simulink model "arduino_lab"  (R2017a)
settings: Solver=VariableStepAuto  StartTime=0.0  StopTime=500  RelTol=1e-3  EnableMultiTasking=on
StartFcn:
  | clear all
libraries: realtime_pacer_lib x1
settings Model: Creator=johnh  LastModifiedBy=John Hedengren
settings OptimizationCC: LifeSpan=inf
settings DebuggingCC: SFUnexpectedBacktrackingDiag=warning  SFNoUnconditionalDefaultTransitionDiag=warning  SFExecutionAtInitializationDiag=none
settings GRTTargetCC: TargetLangStandard=C89/C90 (ANSI)  GeneratePreprocessorConditionals=Disable all
settings ConfigComp: CovMetricSettings=dw  CovHtmlReporting=on  CovSaveCumulativeToWorkspaceVar=on  CovSaveSingleToWorkspaceVar=on  CovExternalEMLEnable=off

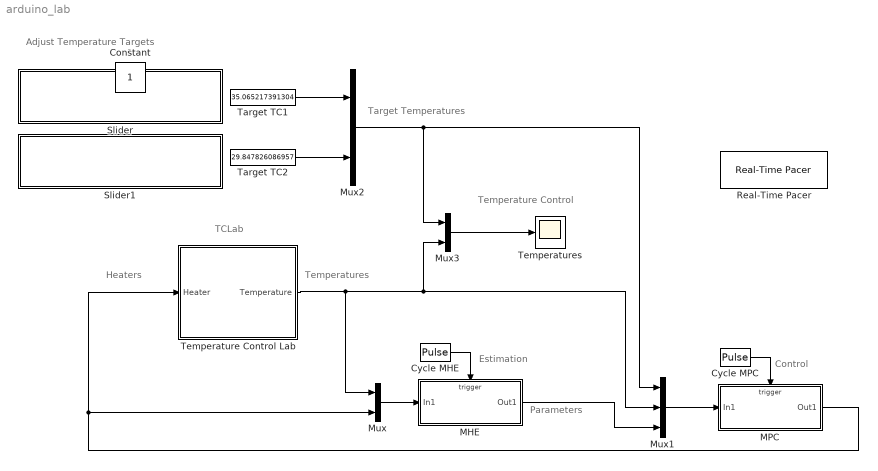
== system arduino_lab ==
  note: Adjust Temperature Targets
  note: Temperature Control
  note: TCLab
  note: Heaters
  note: Estimation
  note: Control
  note: Temperatures
  note: Parameters
  note: Target Temperatures
  Cycle MHE : DiscretePulseGenerator  PulseType=Time based  Period=4  PulseWidth=5
  Cycle MPC : DiscretePulseGenerator  PulseType=Time based  Period=4  PulseWidth=5
  MHE : Subsystem  TreatAsAtomicUnit=on
  MPC : Subsystem  TreatAsAtomicUnit=on
  Mux : Mux  Inputs=2
  Mux1 : Mux  Inputs=3
  Mux2 : Mux  Inputs=2
  Mux3 : Mux  Inputs=2
  Real-Time Pacer : realtime_pacer_lib/Real-Time Pacer  simTimePerRealTime=1
  Slider : Subsystem  DialogController=hmiCreateDDGDialog  IsWebBlock=on  mask(MWDashboardBlock){webBlockId=e384a236-a50c-4b75-ba51-627058c2b810, webBlockType=slider, ShowInLibBrowser=on, ShowInitialText=on, HMISrcModelName=arduino_lab}
      mask prompts: webBlockId "WebBlock Id"; webBlockType "WebBlock Type"; HMISrcModelName "Source Model"
      mask help: SimulinkHMI:dialogs:SliderDialogDesc
      mask Help: helpview([docroot '/mapfiles/simulink.map'], 'hmi_slider')
      mask Display:
      | if strcmp(get_param(bdroot(gcb),'BlockDiagramType'), 'library')
      |     image([(matlabroot) '/toolbox/simulink/hmi/icons/Slider.png']);
      | end
  Slider1 : Subsystem  DialogController=hmiCreateDDGDialog  IsWebBlock=on  mask(MWDashboardBlock){webBlockId=e28f78d7-4053-462e-98b6-be5f9b67005a, webBlockType=slider, ShowInLibBrowser=on, ShowInitialText=on, HMISrcModelName=arduino_lab}
      mask prompts: webBlockId "WebBlock Id"; webBlockType "WebBlock Type"; HMISrcModelName "Source Model"
      mask help: SimulinkHMI:dialogs:SliderDialogDesc
      mask Help: helpview([docroot '/mapfiles/simulink.map'], 'hmi_slider')
      mask Display:
      | if strcmp(get_param(bdroot(gcb),'BlockDiagramType'), 'library')
      |     image([(matlabroot) '/toolbox/simulink/hmi/icons/Slider.png']);
      | end
  Target TC1 : Constant  Value=35.065217391304
  Target TC2 : Constant  Value=29.847826086957
  Temperature Control Lab : Subsystem
      mask Display: image('tclab.png');
  Temperatures : Scope
  1 : Constant  IOType=siggen
  Constant : Constant  IOType=siggen
  wires:
  Cycle MPC/1 -> MPC/Trigger
  MPC/1(Out1) -> Mux/2, Temperature Control Lab/1(Heater)
  Temperature Control Lab/1(Temperature) -> Mux/1, Mux3/2, Mux1/2
  MHE/1(Out1) -> Mux1/3
  Mux/1 -> MHE/1(In1)
  Cycle MHE/1 -> MHE/Trigger
  Mux1/1 -> MPC/1(In1)
  Mux2/1 -> Mux1/1, Mux3/1
  Target TC1/1 -> Mux2/1
  Target TC2/1 -> Mux2/2
  Mux3/1 -> Temperatures/1

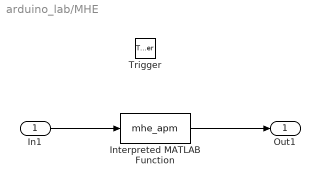
== system arduino_lab/MHE ==
  In1 : Inport  LatchByDelayingOutsideSignal=on
  Trigger : TriggerPort  VariantControl=Variant
  Interpreted MATLAB Function : MATLABFcn  MATLABFcn=mhe_apm  OutputDimensions=5
  Out1 : Outport  InitialOutput=[2.5 5 0.005 0.0025 23]
  wires:
  In1/1 -> Interpreted MATLAB Function/1
  Interpreted MATLAB Function/1 -> Out1/1

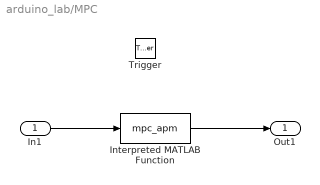
== system arduino_lab/MPC ==
  In1 : Inport  LatchByDelayingOutsideSignal=on
  Trigger : TriggerPort  VariantControl=Variant
  Interpreted MATLAB Function : MATLABFcn  MATLABFcn=mpc_apm  OutputDimensions=2
  Out1 : Outport  InitialOutput=[0 0]
  wires:
  In1/1 -> Interpreted MATLAB Function/1
  Interpreted MATLAB Function/1 -> Out1/1

== system arduino_lab/Slider ==

== system arduino_lab/Slider1 ==

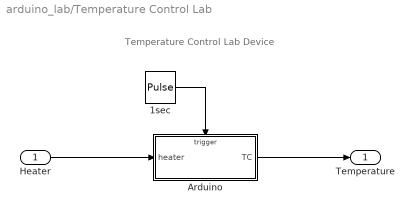
== system arduino_lab/Temperature Control Lab ==
  note: Temperature Control Lab Device
  Heater : Inport
  1sec : DiscretePulseGenerator  PulseType=Time based  Period=1  PulseWidth=50
  Arduino : Subsystem  TreatAsAtomicUnit=on
  Temperature : Outport
  wires:
  1sec/1 -> Arduino/Trigger
  Arduino/1(TC) -> Temperature/1
  Heater/1 -> Arduino/1(heater)

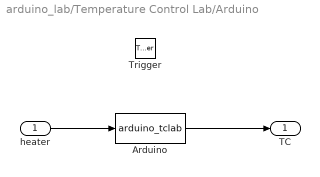
== system arduino_lab/Temperature Control Lab/Arduino ==
  heater : Inport  LatchByDelayingOutsideSignal=on
  Trigger : TriggerPort  VariantControl=Variant
  Arduino : MATLABFcn  MATLABFcn=arduino_tclab
  TC : Outport  InitialOutput=[23 23]
  wires:
  heater/1 -> Arduino/1
  Arduino/1 -> TC/1
